simulink model "sgMdl_IO611_LIN_Loopback"  (R2024b)
settings: Solver=FixedStepAuto  StartTime=0.0  StopTime=inf  RelTol=1e-3  EnableMultiTasking=on
libraries: speedgoatlib_IO611 x7, slrealtimeutilitieslib x2, slrealtimelinlib x2, hdlsllib x1
Description:
  | IO611 - LIN Loopback
settings Model: ModifiedByFormat=Speedgoat  SimulationMode=external  ExtModeEnableFloating=off  ExtModeTrigDuration=100000  Creator=Speedgoat  LastModifiedBy=Speedgoat
settings SolverCC: ConcurrentTasks=on  AlgebraicLoopSolver=TrustRegion  PositivePriorityOrder=on  AutoInsertRateTranBlk=on  InsertRTBMode=Never (minimum delay)
settings DataIOCC: SaveFormat=StructureWithTime
settings OptimizationCC: BlockReduction=off  OptimizeBlockIOStorage=off  BufferReuse=off  GlobalBufferReuse=off  ExpressionFolding=off  LocalBlockOutputs=off  OptimizeDataStoreBuffers=off  BusAssignmentInplaceUpdate=off
settings DebuggingCC: InheritedTsInSrcMsg=none  TasksWithSamePriorityMsg=none  UnconnectedInputMsg=warning  UnconnectedOutputMsg=warning  UnconnectedLineMsg=warning
settings HardwareCC: ProdBitPerLong=64  ProdLongLongMode=on  ProdHWDeviceType=Intel->x86-64 (Linux 64)
settings ModelReferenceCC: EnableRefExpFcnMdlSchedulingChecks=on
settings SFSimCC: CustomCodeUndefinedFunction=UseInterfaceOnly
settings RTWCC: Description=Speedgoat Real-Time Target Machine  SystemTargetFile=speedgoat.tlc  TemplateMakefile=slrealtime_default_tmf  Toolchain=Simulink Real-Time Toolchain  BuildConfiguration=Faster Runs  TargetLang=C++  GPUComputeCapability=3.5  DLArmComputeVersion=19.05
settings SimulinkRealTimeTargetCC: SubcomponentCodeInterfacePackaging=Reusable function  InstructionSetFMA=off  LogToMDFFile=off  SLRTFileLogMaxRuns=10  UseGCCFastMath=on
settings ConfigComp: CovBoundaryAbsTol=1.0e-5

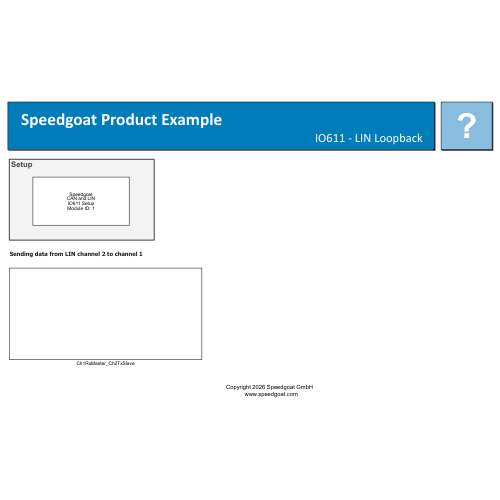
[thumbnail: Simulink's stored preview of the top-level diagram]
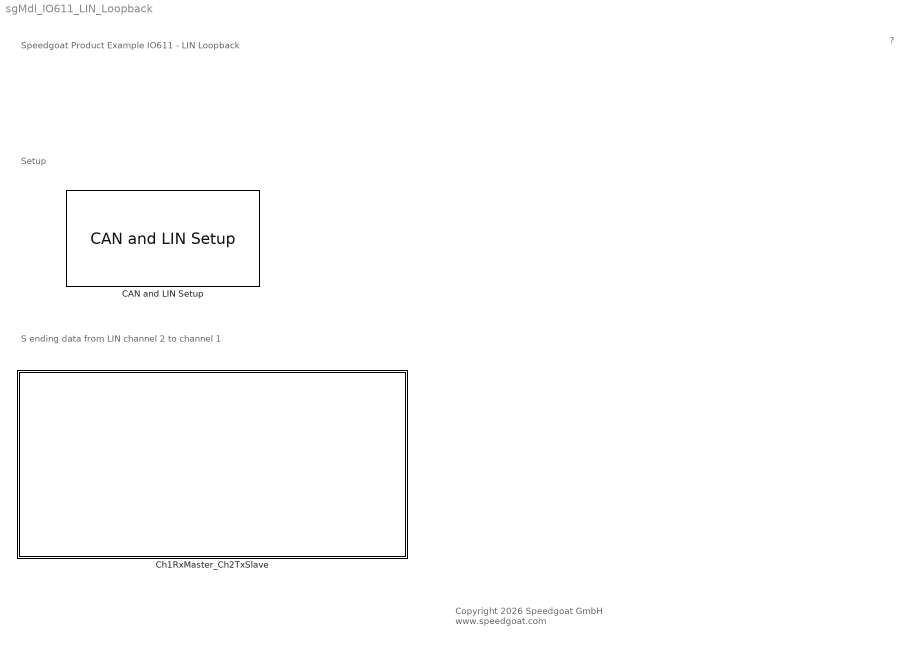
== system sgMdl_IO611_LIN_Loopback ==
  note: S ending data from LIN channel 2 to channel 1
  note: Setup
  note: Speedgoat Product Example
      | IO611 - LIN Loopback
  note: ?
  note: Copyright 2026 Speedgoat GmbH
      |  www.speedgoat.com
  "CAN and LIN Setup " : speedgoatlib_IO611/CAN and LIN Setup   moduleInitValues="[611    1    1   -1   -1]"  id=1  moduleType=IO611  pciSlot=-1  canChn1=Disabled  canChn2=Disabled  canChn3=Disabled  canChn4=Disabled  linChn1=Master  linChn2=Slave  canInitStructArray=[]  canTermStructArray=[]  canChn1InitValues="[1  16   1  31   8   2   1   5   2]"  arbBdrChn1=125 kBaud  arbManBdrChn1=[16,1,31,8]  fdBdrChn1=5.0 MBaud  fdManBdrChn1=[2,1,5,2]  canChn2InitValues="[1   2   1  31   8   2   1   5   2]"  arbBdrChn2=1.0 MBaud  arbManBdrChn2=[2,1,31,8]  fdBdrChn2=5.0 MBaud  fdManBdrChn2=[2,1,5,2]  canChn3InitValues="[1   2   1  31   8   2   1   5   2]"  arbBdrChn3=1.0 MBaud  arbManBdrChn3=[2,1,31,8]  fdBdrChn3=5.0 MBaud  fdManBdrChn3=[2,1,5,2]  canChn4InitValues="[1   2   1  31   8   2   1   5   2]"  arbBdrChn4=1.0 MBaud  arbManBdrChn4=[2,1,31,8]  fdBdrChn4=5.0 MBaud  fdManBdrChn4=[2,1,5,2]  bdrLIN1=19200  linChn1InitValues="[3  19200]"  bdrLIN2=19200  linChn2InitValues="[2  19200]"
      settings: SourceProductName=Simulink Real-Time: Speedgoat I/O Blockset
  Ch1RxMaster_Ch2TxSlave : Subsystem

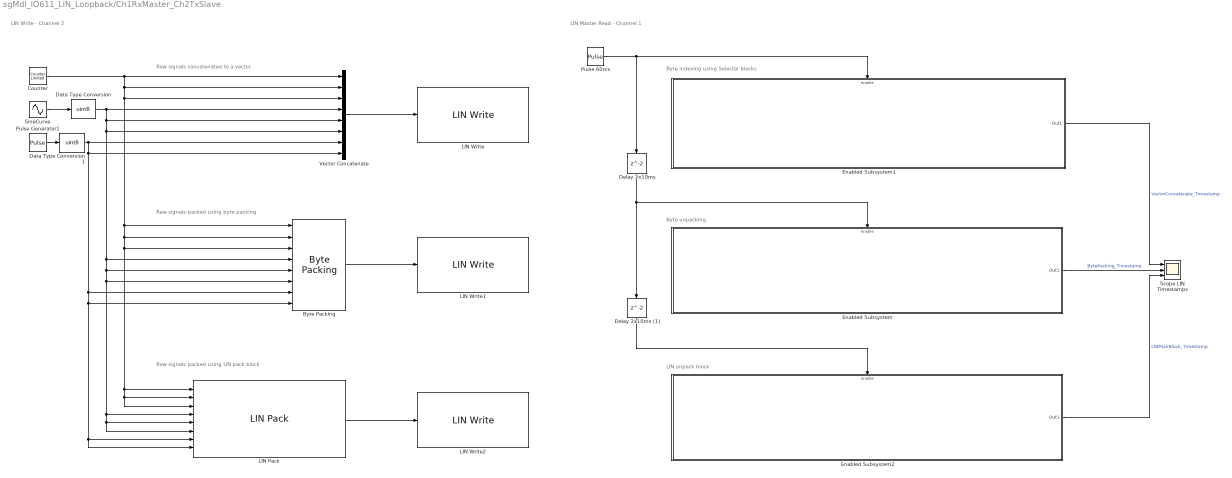
== system sgMdl_IO611_LIN_Loopback/Ch1RxMaster_Ch2TxSlave ==
  note: LIN Write - Channel 2
  note: LIN Master Read - Channel 1
  note: Byte indexing using Selector blocks
  note: Raw signals packed using byte packing
  note: Raw signals concatenated to a vector
  note: Byte unpacking
  note: Raw signals packed using LIN pack block
  note: LIN unpack block
  Byte Packing : slrealtimeutilitieslib/Byte Packing  MaskPackedDataType=uint8  MaskUnpackedDataTypes={'uint8', 'uint8', 'uint8', 'uint8', 'uint8', 'uint8', 'uint8', 'uint8'}  MaskAlignment=1
  Counter : hdlsllib/Sources/Counter Limited  uplimit=255  tsamp=0.01
  Data Type Conversion : DataTypeConversion  OutDataTypeStr=uint8  SaturateOnIntegerOverflow=off  RndMeth=Floor
  Data Type Conversion1 : DataTypeConversion  OutDataTypeStr=uint8  SaturateOnIntegerOverflow=off  RndMeth=Floor
  Delay 2x10ms : Delay  SampleTime=0.01
  Delay 2x10ms (1) : Delay  SampleTime=0.01
  Enabled Subsystem : Subsystem  TreatAsAtomicUnit=on
  Enabled Subsystem1 : Subsystem  TreatAsAtomicUnit=on
  Enabled Subsystem2 : Subsystem  TreatAsAtomicUnit=on
  LIN Pack : slrealtimelinlib/LIN Pack  LDFFileName=IO611_files\LINDescriptorFile.ldf  selectedFrameValue=None  frameId=50
  LIN Write : speedgoatlib_IO611/LIN Write  moduleType=IO611  id=1  channel=2  linType=Slave  messageType=RAW  inputEnableResponse=off  protIdent=48  dlc=8  linVersion=LIN 2.X  defaultMsgData=[1 2 3 4 5 6 7 8]  ts=0.01  initValues=[611 1 0.01 3 2 1 48 8 1 0]
      settings: SourceProductName=Simulink Real-Time: Speedgoat I/O Blockset
  LIN Write1 : speedgoatlib_IO611/LIN Write  moduleType=IO611  id=1  channel=2  linType=Slave  messageType=RAW  inputEnableResponse=off  protIdent=49  dlc=8  linVersion=LIN 2.X  defaultMsgData=[1 2 3 4 5 6 7 8]  ts=0.01  initValues=[611 1 0.01 3 2 1 49 8 1 0]
      settings: SourceProductName=Simulink Real-Time: Speedgoat I/O Blockset
  LIN Write2 : speedgoatlib_IO611/LIN Write  moduleType=IO611  id=1  channel=2  linType=Slave  messageType=RAW  inputEnableResponse=off  protIdent=50  dlc=8  linVersion=LIN 2.X  defaultMsgData=[1 2 3 4 5 6 7 8]  ts=0.01  initValues=[611 1 0.01 3 2 1 50 8 1 0]
      settings: SourceProductName=Simulink Real-Time: Speedgoat I/O Blockset
  Pulse 60ms : DiscretePulseGenerator  Period=6  SampleTime=0.01
  Pulse Generator1 : DiscretePulseGenerator  Amplitude=255  Period=200  PulseWidth=100  SampleTime=0.01
  Scope LIN Timestamps : Scope  NumInputPorts=3
  SineCurve : Sin  Amplitude=127  Bias=128  Frequency=2*pi  SampleTime=0.01
  Vector Concatenate : Concatenate  NumInputs=8
  wires:
  Vector Concatenate/1 -> LIN Write/1
  Data Type Conversion1/1 -> Vector Concatenate/7, LIN Pack/8, LIN Pack/7, Byte Packing/8, Byte Packing/7, Vector Concatenate/8
  Counter/1 -> Vector Concatenate/1, LIN Pack/3, LIN Pack/2, LIN Pack/1, Byte Packing/3, Byte Packing/2, Byte Packing/1, Vector Concatenate/3, Vector Concatenate/2
  SineCurve/1 -> Data Type Conversion/1
  Byte Packing/1 -> LIN Write1/1
  Data Type Conversion/1 -> Vector Concatenate/4, LIN Pack/4, LIN Pack/6, LIN Pack/5, Byte Packing/6, Byte Packing/5, Byte Packing/4, Vector Concatenate/6, Vector Concatenate/5
  Pulse Generator1/1 -> Data Type Conversion1/1
  Pulse 60ms/1 -> Enabled Subsystem1/Enable, Delay 2x10ms/1
  Delay 2x10ms/1 -> Enabled Subsystem/Enable, Delay 2x10ms (1)/1
  Enabled Subsystem/1(Out1) -> Scope LIN Timestamps/2  "BytePacking_Timestamp"
  Enabled Subsystem1/1(Out1) -> Scope LIN Timestamps/1  "VectorConcatenate_Timestamp"
  LIN Pack/1 -> LIN Write2/1
  Enabled Subsystem2/1(Out1) -> Scope LIN Timestamps/3  "LINPackBlock_Timestamp"
  Delay 2x10ms (1)/1 -> Enabled Subsystem2/Enable

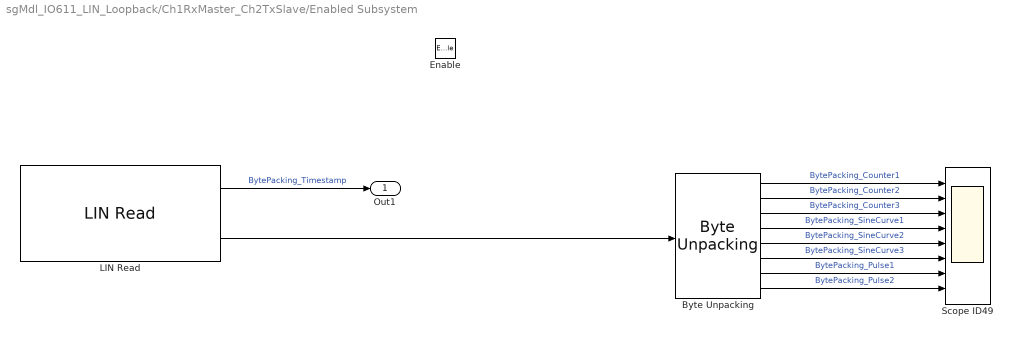
== system sgMdl_IO611_LIN_Loopback/Ch1RxMaster_Ch2TxSlave/Enabled Subsystem ==
  Enable : EnablePort
  Byte Unpacking : slrealtimeutilitieslib/Byte Unpacking  MaskUnpackedDataTypes={'uint8', 'uint8', 'uint8', 'uint8', 'uint8', 'uint8', 'uint8', 'uint8'}  MaskUnpackedDataSizes={[1], [1], [1], [1], [1], [1], [1], [1]}  MaskAlignment=1
  LIN Read : speedgoatlib_IO611/LIN Read  moduleType=IO611  id=1  channel=1  linType=Master  messageType=RAW  protIdent=49  dlc=8  linVersion=LIN 2.X  enaUpdateState=off  enaMsgType=off  enaDataOverrun=off  enaTimeStamp=on  ts=0.01  initValues=[611 1 0.01 2 2 0 49 8 1 0 0 0 1]
      settings: SourceProductName=Simulink Real-Time: Speedgoat I/O Blockset
  Scope ID49 : Scope  NumInputPorts=8
  Out1 : Outport
  wires:
  Byte Unpacking/8 -> Scope ID49/8  "BytePacking_Pulse2"
  Byte Unpacking/6 -> Scope ID49/6  "BytePacking_SineCurve3"
  Byte Unpacking/7 -> Scope ID49/7  "BytePacking_Pulse1"
  Byte Unpacking/5 -> Scope ID49/5  "BytePacking_SineCurve2"
  LIN Read/2 -> Byte Unpacking/1
  Byte Unpacking/1 -> Scope ID49/1  "BytePacking_Counter1"
  Byte Unpacking/2 -> Scope ID49/2  "BytePacking_Counter2"
  Byte Unpacking/3 -> Scope ID49/3  "BytePacking_Counter3"
  LIN Read/1 -> Out1/1  "BytePacking_Timestamp"
  Byte Unpacking/4 -> Scope ID49/4  "BytePacking_SineCurve1"

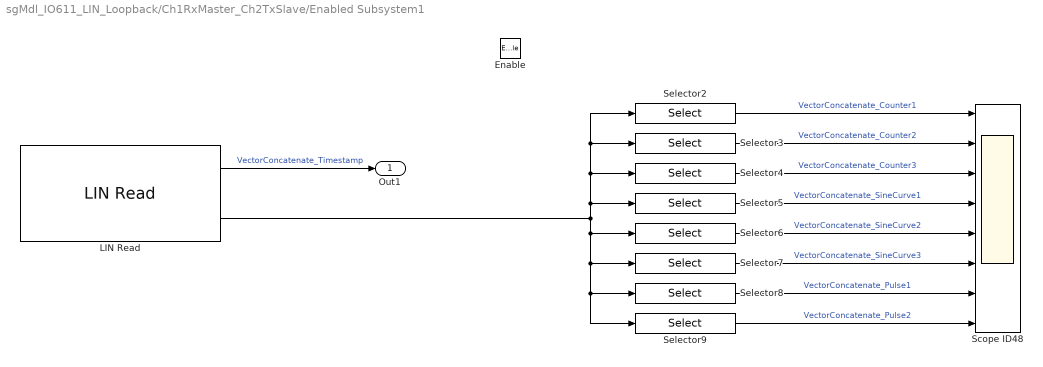
== system sgMdl_IO611_LIN_Loopback/Ch1RxMaster_Ch2TxSlave/Enabled Subsystem1 ==
  Enable : EnablePort
  LIN Read : speedgoatlib_IO611/LIN Read  moduleType=IO611  id=1  channel=1  linType=Master  messageType=RAW  protIdent=48  dlc=8  linVersion=LIN 2.X  enaUpdateState=off  enaMsgType=off  enaDataOverrun=off  enaTimeStamp=on  ts=0.01  initValues=[611 1 0.01 2 2 0 48 8 1 0 0 0 1]
      settings: SourceProductName=Simulink Real-Time: Speedgoat I/O Blockset
  Scope ID48 : Scope  NumInputPorts=8
  Selector2 : Selector  InputPortWidth=8  IndexOptions=Index vector (dialog)  Indices=[1]  OutputSizes=1
  Selector3 : Selector  InputPortWidth=8  IndexOptions=Index vector (dialog)  Indices=[2]  OutputSizes=1
  Selector4 : Selector  InputPortWidth=8  IndexOptions=Index vector (dialog)  Indices=[3]  OutputSizes=1
  Selector5 : Selector  InputPortWidth=8  IndexOptions=Index vector (dialog)  Indices=[4]  OutputSizes=1
  Selector6 : Selector  InputPortWidth=8  IndexOptions=Index vector (dialog)  Indices=[5]  OutputSizes=1
  Selector7 : Selector  InputPortWidth=8  IndexOptions=Index vector (dialog)  Indices=[6]  OutputSizes=1
  Selector8 : Selector  InputPortWidth=8  IndexOptions=Index vector (dialog)  Indices=[7]  OutputSizes=1
  Selector9 : Selector  InputPortWidth=8  IndexOptions=Index vector (dialog)  Indices=[8]  OutputSizes=1
  Out1 : Outport
  wires:
  Selector5/1 -> Scope ID48/4  "VectorConcatenate_SineCurve1"
  Selector9/1 -> Scope ID48/8  "VectorConcatenate_Pulse2"
  Selector6/1 -> Scope ID48/5  "VectorConcatenate_SineCurve2"
  Selector3/1 -> Scope ID48/2  "VectorConcatenate_Counter2"
  Selector8/1 -> Scope ID48/7  "VectorConcatenate_Pulse1"
  LIN Read/2 -> Selector5/1, Selector4/1, Selector2/1, Selector3/1, Selector9/1, Selector8/1, Selector7/1, Selector6/1
  Selector4/1 -> Scope ID48/3  "VectorConcatenate_Counter3"
  Selector2/1 -> Scope ID48/1  "VectorConcatenate_Counter1"
  Selector7/1 -> Scope ID48/6  "VectorConcatenate_SineCurve3"
  LIN Read/1 -> Out1/1  "VectorConcatenate_Timestamp"

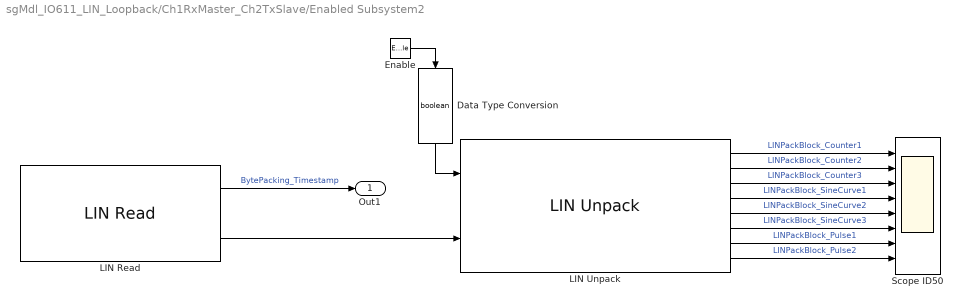
== system sgMdl_IO611_LIN_Loopback/Ch1RxMaster_Ch2TxSlave/Enabled Subsystem2 ==
  Enable : EnablePort  ShowOutputPort=on
  Data Type Conversion : DataTypeConversion  OutDataTypeStr=boolean  SaturateOnIntegerOverflow=off  RndMeth=Floor
  LIN Read : speedgoatlib_IO611/LIN Read  moduleType=IO611  id=1  channel=1  linType=Master  messageType=RAW  protIdent=50  dlc=8  linVersion=LIN 2.X  enaUpdateState=off  enaMsgType=off  enaDataOverrun=off  enaTimeStamp=on  ts=0.01  initValues=[611 1 0.01 2 2 0 50 8 1 0 0 0 1]
      settings: SourceProductName=Simulink Real-Time: Speedgoat I/O Blockset
  LIN Unpack : slrealtimelinlib/LIN Unpack  LDFFileName=IO611_files\LINDescriptorFile.ldf  selectedFrameValue=None  frameId=50
  Scope ID50 : Scope  NumInputPorts=8
  Out1 : Outport
  wires:
  LIN Unpack/8 -> Scope ID50/8  "LINPackBlock_Pulse2"
  LIN Unpack/6 -> Scope ID50/6  "LINPackBlock_SineCurve3"
  LIN Unpack/7 -> Scope ID50/7  "LINPackBlock_Pulse1"
  LIN Unpack/5 -> Scope ID50/5  "LINPackBlock_SineCurve2"
  LIN Read/2 -> LIN Unpack/2
  LIN Unpack/1 -> Scope ID50/1  "LINPackBlock_Counter1"
  LIN Unpack/2 -> Scope ID50/2  "LINPackBlock_Counter2"
  LIN Unpack/3 -> Scope ID50/3  "LINPackBlock_Counter3"
  LIN Read/1 -> Out1/1  "BytePacking_Timestamp"
  LIN Unpack/4 -> Scope ID50/4  "LINPackBlock_SineCurve1"
  Enable/1 -> Data Type Conversion/1
  Data Type Conversion/1 -> LIN Unpack/1
